simulink model "sampleModel1464"  (R2023a)
settings: Solver=VariableStepAuto  StartTime=0.0  StopTime=10.0  RelTol=1e-3
libraries: hdlsllib x6, simulink x4
settings Model: Creator=user1  LastModifiedBy=user1

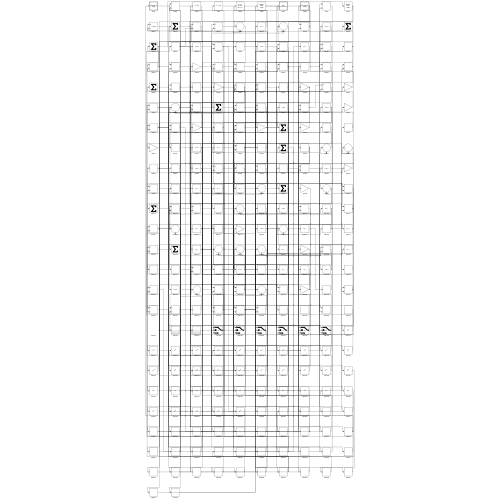
[thumbnail: Simulink's stored preview of the top-level diagram]
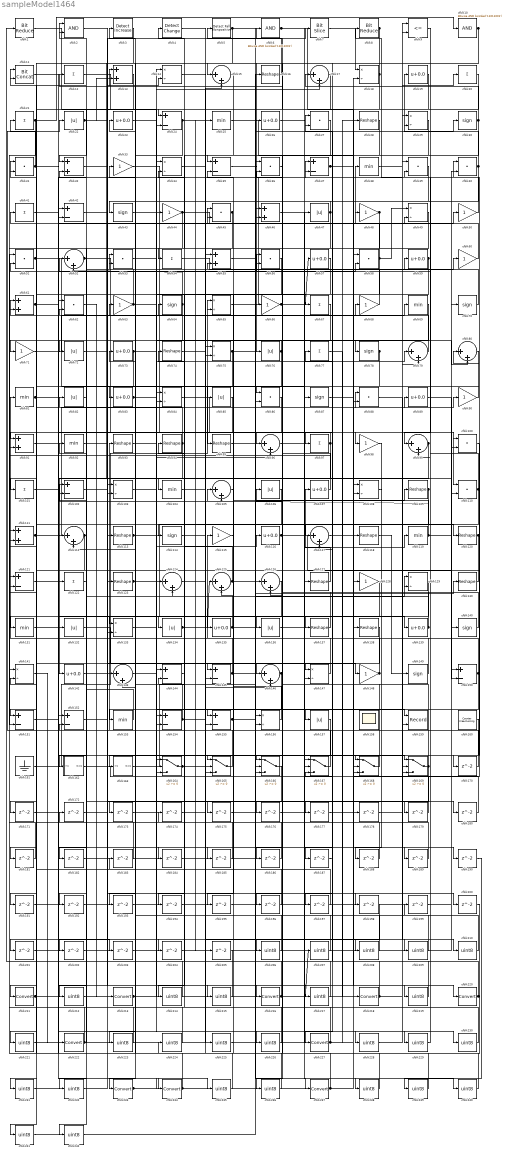
== system sampleModel1464 ==
  cfblk1 : hdlsllib/Logic and Bit Operations/Bit Reduce  mode=AND
  cfblk10 : simulink/Logic and Bit Operations/Bitwise Operator  logicop=AND  UseBitMask=on  BitMask=bin2dec('11011001')  BitMaskRealWorld=Stored Integer
      settings: LibrarySourceBlock=|
      | hdlsllib/Logic and Bit
      | Operations/Bitwise
      | Operator
  cfblk{27,31,36,39..40,45,51,53,56,58,62,86,88,100,110} (15 alike) : DotProduct  OutDataTypeStr=Inherit: Inherit via internal rule
  cfblk{12,20..21,41,54,67,77,97,101,122} (10 alike) : Sum  Inputs=+
  cfblk{24,35,37,42,102,121,144..145,150..152,154..155} (13 alike) : Sum  Inputs=+-
  cfblk{14,18,29,34,49,65,75,84,103,108,129,133,141,147,156} (15 alike) : Product  Inputs=*/  RndMeth=Zero  SaturateOnIntegerOverflow=on
  cfblk{25,38,69,81,92,104,119,131,153} (9 alike) : MinMax
  cfblk{15,17,52,79..80,96,99,105,112,117,124..126,143,146} (15 alike) : Sum  Inputs=|++
  cfblk{22,47,72,76,82,85,106,132,134,136,157} (11 alike) : Abs  SaturateOnIntegerOverflow=off
  cfblk{19,23,26,57,59,73,83,89,107,116,135,139,142} (13 alike) : Bias  Bias=0.0  SaturateOnIntegerOverflow=off
  cfblk{16,28,74,93..95,109,113,118,120,123,127,130,137..138} (15 alike) : Reshape
  cfblk11 : hdlsllib/Logic and Bit Operations/Bit Concat  numInputs=2
  cfblk{13,32,46,55,61,91,111} (7 alike) : Sum
  cfblk{30,43,64,70,78,87,114,140,149} (9 alike) : Signum
  cfblk{33,44,48,50,60,63,66,68,71,90,98,115,128,148} (14 alike) : Gain
  cfblk158 : Scope
      settings: Floating=on
  cfblk159 : Record  FileSettingsInternal="{\"entries\":[{\"content\":{\"excelSettings\":{\"content\":{},\"type\":\"Streamout.ExcelSettings\"}},\"type\":\"Streamout.FileSettingStorage\",\"uuid\":\"\"}],\"packageUris\":[\"http:\\/\\/schema.mathworks.com\\/mf0\\/streamout_blocks\\/R2020a\"],\"version\":\"1.0\"}"  Layout=[1 1]  SignalsInternal="{\"entries\":[{\"content\":{\"signals\":[{\"content\":{\"blockPath\":[],\"dimensions\":[1],\"domain\":\"\",\"lineColor\":\"#a2142f\",\"plots\":[1],\"port\":1,\"signalID\":864,\"signalName\":\"XY Graph:1\"},\"type\":\"RecordBlkView.Signal\",\"uuid\":\"\"},{\"content\":{\"blockPath\":[],\"dimensions\":[1],\"domain\":\"\",\"lineColor\":\"#139fff\",\"plots\":[1],\"port\":2,\"signalID\":867,\"signalName\":\"XY Graph:2\"},\"type\":\"RecordBlkView.Signal\",\"uuid\":\"\"}]},\"type\":\"RecordBlkView.InputSignals\",\"uuid\":\"\"}],\"packageUris\":[\"http:\\/\\/schema.mathworks.com\\/mf0\\/streamout_blocks\\/R2020a\"],\"version\":\"1.0\"}"  VisualizationBindings="{\"xyplotplugin\":{\"info\":[{\"series\":[{\"bindingParametersList\":[{\"parameter\":\"X-Axis\",\"signalID\":864,\"signalName\":\"XY Graph:1\"},{\"parameter\":\"Y-Axis\",\"signalID\":867,\"signalName\":\"XY Graph:2\"}],\"seriesID\":36667}],\"subplotID\":1}]}}"  CompatibilityTag=XY  st=-1
  cfblk160 : hdlsllib/Sources/Counter Free-Running  NumBits=16  tsamp=-1
  cfblk161 : Ground
  cfblk162 : Subsystem
      settings: LibrarySourceBlock=|
      | hdlsllib/Ports &
      | Subsystems/Subsystem
  cfblk163 : Subsystem
      settings: LibrarySourceBlock=|
      | hdlsllib/Ports &
      | Subsystems/Subsystem
  cfblk{164..169} (6 alike) : Switch  SaturateOnIntegerOverflow=off  InputSameDT=off
  cfblk{170..205} (36 alike) : Delay  SampleTime=1
  cfblk2 : Logic  AllPortsSameDT=off  OutDataTypeStr=boolean
  cfblk{206..210,212,214..215,217,219,221,223..226,228..232,235..236,238..242} (27 alike) : DataTypeConversion  OutDataTypeStr=uint8  SaturateOnIntegerOverflow=off  RndMeth=Floor
  cfblk{211,213,216,218,220,222,227,233..234,237} (10 alike) : DataTypeConversion  SaturateOnIntegerOverflow=off  RndMeth=Floor
  cfblk3 : simulink/Logic and Bit Operations/Detect Increase  vinit=0.0  OutDataTypeStr=boolean
      settings: LibrarySourceBlock=|
      | hdlsllib/Logic and Bit
      | Operations/Detect
      | Increase
  cfblk4 : simulink/Logic and Bit Operations/Detect Change  vinit=0  OutDataTypeStr=boolean
      settings: LibrarySourceBlock=|
      | hdlsllib/Logic and Bit
      | Operations/Detect
      | Change
  cfblk5 : hdlsllib/Logic and Bit Operations/Detect Fall Nonpositive  vinit=0  OutDataTypeStr=boolean
  cfblk6 : simulink/Logic and Bit Operations/Bitwise Operator  logicop=AND  UseBitMask=on  BitMask=bin2dec('11011001')  BitMaskRealWorld=Stored Integer
      settings: LibrarySourceBlock=|
      | hdlsllib/Logic and Bit
      | Operations/Bitwise
      | Operator
  cfblk7 : hdlsllib/Logic and Bit Operations/Bit Slice  lidx=7  ridx=0
  cfblk8 : hdlsllib/Logic and Bit Operations/Bit Reduce  mode=AND
  cfblk9 : RelationalOperator  Operator=<=  OutDataTypeStr=boolean  InputSameDT=off
  wires:
  cfblk145/1 -> cfblk81/1, cfblk60/1
  cfblk169/1 -> cfblk13/1, cfblk196/1
  cfblk118/1 -> cfblk149/1
  cfblk156/1 -> cfblk45/1
  cfblk3/1 -> cfblk104/1
  cfblk76/1 -> cfblk72/1, cfblk221/1
  cfblk167/1 -> cfblk22/1
  cfblk165/1 -> cfblk93/1
  cfblk52/1 -> cfblk98/1, cfblk14/2
  cfblk164/1 -> cfblk94/1, cfblk37/2
  cfblk154/1 -> cfblk25/1, cfblk112/2
  cfblk31/1 -> cfblk21/1, cfblk139/1
  cfblk99/1 -> cfblk142/1, cfblk136/1
  cfblk33/1 -> cfblk110/1
  cfblk161/1 -> cfblk65/1
  cfblk141/1 -> cfblk222/1
  cfblk121/1 -> cfblk234/1
  cfblk21/1 -> cfblk10/1, cfblk61/2
  cfblk84/1 -> cfblk96/1
  cfblk5/1 -> cfblk71/1, cfblk180/1
  cfblk56/1 -> cfblk134/1
  cfblk20/1 -> cfblk32/1
  cfblk10/1 -> cfblk76/1, cfblk26/1
  cfblk19/1 -> cfblk42/2
  cfblk40/1 -> cfblk19/1, cfblk164/3
  cfblk71/1 -> cfblk68/1
  cfblk147/1 -> cfblk115/1
  cfblk125/1 -> cfblk64/1, cfblk167/2
  cfblk90/1 -> cfblk86/1
  cfblk162/1(Out1) -> cfblk80/1
  cfblk66/1 -> cfblk57/1, cfblk80/2
  cfblk77/1 -> cfblk218/1
  cfblk62/1 -> cfblk213/1
  cfblk134/1 -> cfblk125/1, cfblk90/1
  cfblk115/1 -> cfblk135/1
  cfblk87/1 -> cfblk220/1
  cfblk78/1 -> cfblk137/1, cfblk114/1, cfblk187/1
  cfblk94/1 -> cfblk31/1, cfblk154/2
  cfblk41/1 -> cfblk110/2
  cfblk127/1 -> cfblk107/1
  cfblk57/1 -> cfblk145/1
  cfblk120/1 -> cfblk40/1, cfblk159/2
  cfblk49/1 -> cfblk146/1
  cfblk39/1 -> cfblk227/1
  cfblk16/1 -> cfblk5/1
  cfblk51/1 -> cfblk127/1, cfblk169/1
  cfblk83/1 -> cfblk153/1, cfblk96/2
  cfblk113/1 -> cfblk120/1, cfblk166/3
  cfblk148/1 -> cfblk63/1, cfblk3/1
  cfblk96/1 -> cfblk47/1
  cfblk101/1 -> cfblk132/1
  cfblk64/1 -> cfblk143/2, cfblk52/2
  cfblk15/1 -> cfblk35/1
  cfblk1/1 -> cfblk144/1
  cfblk67/1 -> cfblk133/1
  cfblk155/1 -> cfblk109/1, cfblk129/2, cfblk169/2, cfblk238/1
  cfblk29/1 -> cfblk157/1
  cfblk160/1 -> cfblk233/1
  cfblk109/1 -> cfblk105/2, cfblk194/1
  cfblk89/1 -> cfblk140/1
  cfblk130/1 -> cfblk122/1
  cfblk92/1 -> cfblk216/1
  cfblk136/1 -> cfblk119/1
  cfblk86/1 -> cfblk155/1
  cfblk60/1 -> cfblk38/1
  cfblk116/1 -> cfblk150/2, cfblk168/3
  cfblk132/1 -> cfblk156/1
  cfblk25/1 -> cfblk138/1
  cfblk80/1 -> cfblk95/1
  cfblk168/1 -> cfblk27/1
  cfblk65/1 -> cfblk9/2
  cfblk32/1 -> cfblk113/1
  cfblk135/1 -> cfblk2/1, cfblk129/1, cfblk45/2, cfblk29/2
  cfblk149/1 -> cfblk53/1
  cfblk35/1 -> cfblk66/1
  cfblk7/1 -> cfblk18/1
  cfblk6/1 -> cfblk108/2, cfblk198/1
  cfblk24/1 -> cfblk146/2, cfblk83/1, cfblk205/1
  cfblk139/1 -> cfblk12/1, cfblk124/2
  cfblk68/1 -> cfblk23/1
  cfblk102/1 -> cfblk123/1
  cfblk61/1 -> cfblk49/2, cfblk184/1, cfblk185/1
  cfblk73/1 -> cfblk44/1, cfblk112/1
  cfblk37/1 -> cfblk100/1, cfblk117/2
  cfblk79/1 -> cfblk32/2
  cfblk108/1 -> cfblk168/1
  cfblk95/1 -> cfblk147/1
  cfblk137/1 -> cfblk61/1
  cfblk8/1 -> cfblk97/1, cfblk193/1
  cfblk111/1 -> cfblk88/1, cfblk203/1
  cfblk163/1(Out1) -> cfblk130/1
  cfblk9/1 -> cfblk99/1
  cfblk30/1 -> cfblk17/1, cfblk236/1
  cfblk70/1 -> cfblk41/1
  cfblk146/1 -> cfblk156/2, cfblk186/1
  cfblk128/1 -> cfblk211/1
  cfblk142/1 -> cfblk7/1
  cfblk50/1 -> cfblk8/1
  cfblk150/1 -> cfblk163/1(In1), cfblk105/1
  cfblk54/1 -> cfblk59/1
  cfblk58/1 -> cfblk131/1, cfblk11/2, cfblk49/1
  cfblk119/1 -> cfblk70/1, cfblk35/2
  cfblk28/1 -> cfblk166/1
  cfblk63/1 -> cfblk11/1, cfblk78/1
  cfblk152/1 -> cfblk89/1
  cfblk59/1 -> cfblk75/2, cfblk197/1
  cfblk12/1 -> cfblk154/1
  cfblk38/1 -> cfblk20/1
  cfblk114/1 -> cfblk147/2
  cfblk55/1 -> cfblk237/1
  cfblk124/1 -> cfblk50/1
  cfblk93/1 -> cfblk159/1
  cfblk75/1 -> cfblk16/1, cfblk30/1, cfblk169/3, cfblk165/2
  cfblk82/1 -> cfblk52/1
  cfblk27/1 -> cfblk54/1
  cfblk43/1 -> cfblk85/1
  cfblk44/1 -> cfblk101/1, cfblk48/1
  cfblk117/1 -> cfblk69/1
  cfblk140/1 -> cfblk102/1
  cfblk123/1 -> cfblk167/1, cfblk124/1, cfblk17/2
  cfblk81/1 -> cfblk37/1, cfblk58/2
  cfblk107/1 -> cfblk6/1
  cfblk153/1 -> cfblk2/2
  cfblk133/1 -> cfblk79/1
  cfblk18/1 -> cfblk15/1, cfblk24/1
  cfblk22/1 -> cfblk148/1, cfblk13/2, cfblk165/3
  cfblk53/1 -> cfblk67/1
  cfblk143/1 -> cfblk116/1
  cfblk45/1 -> cfblk151/2, cfblk173/1
  cfblk97/1 -> cfblk91/1, cfblk91/2, cfblk192/1
  cfblk129/1 -> cfblk165/1
  cfblk110/1 -> cfblk117/1, cfblk51/2
  cfblk112/1 -> cfblk151/1, cfblk202/1, cfblk242/1
  cfblk131/1 -> cfblk56/1
  cfblk47/1 -> cfblk126/2, cfblk43/1
  cfblk11/1 -> cfblk100/2
  cfblk48/1 -> cfblk162/1(In1), cfblk232/1
  cfblk100/1 -> cfblk170/1
  cfblk170/1 -> cfblk144/2
  cfblk69/1 -> cfblk171/1
  cfblk172/1 -> cfblk143/1
  cfblk173/1 -> cfblk15/2
  cfblk2/1 -> cfblk175/1
  cfblk157/1 -> cfblk176/1
  cfblk176/1 -> cfblk18/2
  cfblk74/1 -> cfblk177/1
  cfblk177/1 -> cfblk88/2
  cfblk178/1 -> cfblk79/2
  cfblk23/1 -> cfblk179/1
  cfblk179/1 -> cfblk9/1
  cfblk180/1 -> cfblk168/2
  cfblk106/1 -> cfblk181/1
  cfblk181/1 -> cfblk51/1
  cfblk166/1 -> cfblk182/1
  cfblk182/1 -> cfblk126/1
  cfblk183/1 -> cfblk31/2
  cfblk184/1 -> cfblk75/1
  cfblk185/1 -> cfblk152/2
  cfblk186/1 -> cfblk102/2
  cfblk187/1 -> cfblk167/3
  cfblk98/1 -> cfblk188/1
  cfblk188/1 -> cfblk27/2
  cfblk14/1 -> cfblk189/1
  cfblk189/1 -> cfblk125/2
  cfblk34/1 -> cfblk190/1
  cfblk13/1 -> cfblk191/1
  cfblk191/1 -> cfblk155/2
  cfblk192/1 -> cfblk164/1
  cfblk193/1 -> cfblk56/2
  cfblk194/1 -> cfblk108/1
  cfblk105/1 -> cfblk195/1
  cfblk195/1 -> cfblk40/2
  cfblk196/1 -> cfblk164/2
  cfblk197/1 -> cfblk111/2
  cfblk199/1 -> cfblk99/2
  cfblk72/1 -> cfblk200/1
  cfblk138/1 -> cfblk201/1
  cfblk201/1 -> cfblk145/2
  cfblk202/1 -> cfblk133/2
  cfblk203/1 -> cfblk84/2
  cfblk85/1 -> cfblk204/1
  cfblk204/1 -> cfblk150/1
  cfblk205/1 -> cfblk1/1
  cfblk36/1 -> cfblk206/1
  cfblk206/1 -> cfblk65/2
  cfblk207/1 -> cfblk36/1
  cfblk175/1 -> cfblk208/1
  cfblk208/1 -> cfblk36/2
  cfblk4/1 -> cfblk209/1
  cfblk209/1 -> cfblk73/1
  cfblk88/1 -> cfblk210/1
  cfblk210/1 -> cfblk4/1
  cfblk211/1 -> cfblk24/2, cfblk84/1
  cfblk122/1 -> cfblk212/1
  cfblk212/1 -> cfblk128/1
  cfblk213/1 -> cfblk207/1, cfblk29/1
  cfblk144/1 -> cfblk214/1
  cfblk214/1 -> cfblk62/1
  cfblk171/1 -> cfblk215/1
  cfblk215/1 -> cfblk62/2
  cfblk216/1 -> cfblk178/1, cfblk74/1
  cfblk42/1 -> cfblk217/1
  cfblk217/1 -> cfblk92/1
  cfblk218/1 -> cfblk14/1, cfblk34/1
  cfblk26/1 -> cfblk219/1
  cfblk219/1 -> cfblk77/1
  cfblk220/1 -> cfblk199/1, cfblk33/1
  cfblk221/1 -> cfblk87/1
  cfblk222/1 -> cfblk172/1, cfblk111/1
  cfblk126/1 -> cfblk223/1
  cfblk223/1 -> cfblk141/1
  cfblk200/1 -> cfblk224/1
  cfblk224/1 -> cfblk141/2
  cfblk174/1 -> cfblk225/1
  cfblk225/1 -> cfblk58/1
  cfblk151/1 -> cfblk226/1
  cfblk226/1 -> cfblk174/1
  cfblk227/1 -> cfblk34/2, cfblk28/1, cfblk82/1
  cfblk104/1 -> cfblk228/1
  cfblk228/1 -> cfblk39/1
  cfblk91/1 -> cfblk229/1
  cfblk229/1 -> cfblk39/2
  cfblk103/1 -> cfblk230/1
  cfblk230/1 -> cfblk53/2
  cfblk198/1 -> cfblk231/1
  cfblk231/1 -> cfblk103/1
  cfblk232/1 -> cfblk103/2
  cfblk233/1 -> cfblk118/1, cfblk235/1
  cfblk234/1 -> cfblk86/2, cfblk42/1
  cfblk235/1 -> cfblk121/1
  cfblk236/1 -> cfblk121/2
  cfblk237/1 -> cfblk183/1, cfblk152/1, cfblk166/2
  cfblk238/1 -> cfblk55/1
  cfblk190/1 -> cfblk239/1
  cfblk239/1 -> cfblk55/2
  cfblk46/1 -> cfblk240/1
  cfblk240/1 -> cfblk106/1
  cfblk17/1 -> cfblk241/1
  cfblk241/1 -> cfblk46/1
  cfblk242/1 -> cfblk46/2

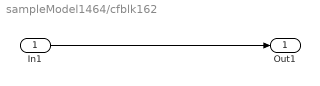
== system sampleModel1464/cfblk162 ==
  In1 : Inport
  Out1 : Outport
  wires:
  In1/1 -> Out1/1

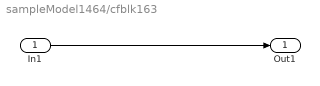
== system sampleModel1464/cfblk163 ==
  In1 : Inport
  Out1 : Outport
  wires:
  In1/1 -> Out1/1
